simulink model "a8_real_control_smc"  (R2023b)
settings: Solver=FixedStepAuto  StartTime=0.0  StopTime=inf  RelTol=1e-3
undefined symbols (not defined in the file): dev, Main, pid_y_i, pwm_output0
libraries: simulink x15, slpidlib x6, px4Sensorslib x5, px4lib x1, px4uORBlib x1
(part 2 of 2)

== system a8_real_control_smc/RC_cmd/RC2FlightMode/If Action Subsystem2 ==
  In1 : Inport
  Action Port : ActionPort  ActionPortLabel=else
  Out1 : Outport
  wires:
  In1/1 -> Out1/1

== matlab function a8_real_control_smc/Subsystem2/MATLAB Function4 ==
  data: dt input; e_psi input double; u4 output double; e_psi_dot input double; psi_des_dotdot input; s_psi_integ input; phi_dot input; theta_dot input; psi_dot input; reset input; s output; s_psi_integ output
function [u4, s, s_psi_integ] = u4fcn(dt, e_psi, e_psi_dot, psi_des_dotdot,...
                    s_psi_integ, phi_dot, theta_dot, psi_dot, reset)

if (reset == 1); s_psi_integ = 0; end
m = 0.67; g = 9.80665; Ix = 0.0035; Iy = 0.0035; Iz = 0.0069; L = 0.25 / 2;
Kpsi = 0;

alpha = 2;beta = 1;gamma = 0.4;
mu = 25/17;r = 1.5;
K = 5; K1 = 1.5; K2 = 1;

s = alpha * e_psi +  real(beta * sign(e_psi_dot) * (abs(e_psi_dot)) ^ mu) + real(gamma * sign(e_psi) * (abs(e_psi)) ^ r);
s_psi_integ = s_psi_integ + K2 * sign(s) * dt;
s_integ_max = 2;
if s_psi_integ > s_integ_max
    s_psi_integ = s_integ_max;
elseif s_psi_integ < -s_integ_max
    s_psi_integ = -s_integ_max;
end

u4 = -Iz*((Ix-Iy)/Iz*phi_dot*theta_dot - Kpsi/Iz*psi_dot - psi_des_dotdot + alpha/(beta*mu)*sign(e_psi_dot) * (abs(e_psi_dot))^(2-mu)...
    + gamma*r/(beta*mu)*(sign(e_psi) * (abs(e_psi))^(r-1))* sign(e_psi_dot) * (abs(e_psi_dot))^(2-mu) + K1*(abs(s))^(1/2)*sign(s)...
    + s_psi_integ);
u4 = u4 * K;

== matlab function a8_real_control_smc/Subsystem2/MATLAB Function1 ==
  data: dt input; e_theta input double; u3 output double; e_theta_dot input double; theta_des_dotdot input; s_theta_integ input; phi_dot input; theta_dot input; psi_dot input; reset input; s output; s_theta_integ output
function [u3, s, s_theta_integ] = u3fcn(dt, e_theta, e_theta_dot, theta_des_dotdot,...
                    s_theta_integ, phi_dot, theta_dot, psi_dot, reset)

if (reset == 1); s_theta_integ = 0; end
m = 0.67; g = 9.80665; Ix = 0.0035; Iy = 0.0035; Iz = 0.0069; L = 0.25 / 2;
Ktheta = 0;

alpha = 2;beta = 1;gamma = 0.4;
mu = 27/17;r = 1.5;
K1 = 1.5; K2 = (K1^2)/2;

s = alpha * e_theta +  (beta * sign(e_theta_dot) * (abs(e_theta_dot)) ^ mu) + (gamma * sign(e_theta) * (abs(e_theta)) ^ r);
s_theta_integ = s_theta_integ + K2 * sign(s) * dt;
s_integ_max = 2;
if s_theta_integ > s_integ_max
    s_theta_integ = s_integ_max;
elseif s_theta_integ < -s_integ_max
    s_theta_integ = -s_integ_max;
end

u3 = -Iy*((Iz-Ix)/Iy*phi_dot*psi_dot - Ktheta/Iy*theta_dot - theta_des_dotdot + alpha/(beta*mu)*sign(e_theta_dot) * (abs(e_theta_dot))^(2-mu)...
    + gamma*r/(beta*mu)*(sign(e_theta) * (abs(e_theta))^(r-1))* sign(e_theta_dot) * (abs(e_theta_dot))^(2-mu) + K1*(abs(s))^(1/2)*sign(s)...
    + s_theta_integ);

== matlab function a8_real_control_smc/quat2eul ==
  data: q input; phi output; theta output; psi output
function [phi,theta,psi] = quat2eul(q)

% Quaternion conversion to Euler angles based on the PX4 Firmware v1.10.2
% release.

phi = atan2(2*(q(1)*q(2) + q(3)* q(4)), q(1)^2 - q(2)^2 - q(3)^2 + q(4)^2);
theta = asin(-2*(q(2)*q(4) - q(1)*q(3)));
psi = atan2(2*(q(2)*q(3) + q(1)* q(4)), q(1)^2 + q(2)^2 - q(3)^2 - q(4)^2);

end

== matlab function a8_real_control_smc/Subsystem1/MATLAB Function1 ==
  data: phi input double; gain output double; theta input double
function gain = fcn(phi, theta)

gain = 1/(cos(phi) * cos(theta));

== matlab function a8_real_control_smc/Subsystem2/MATLAB Function2 ==
  data: dt input; e_phi input double; u2 output double; e_phi_dot input double; phi_des_dotdot input; s_phi_integ input; phi_dot input; theta_dot input; psi_dot input; s_integ_max input; alpha input; beta input; gamma input; mu input; r input; K1 input; K2 input; reset input; s output; s_phi_integ output
function [u2, s, s_phi_integ] = u2fcn(dt, e_phi, e_phi_dot, phi_des_dotdot,...
                    s_phi_integ, phi_dot, theta_dot, psi_dot, s_integ_max, ...
                    alpha, beta, gamma, mu ,r , K1, K2, reset)

if (reset == 1); s_phi_integ = 0; end
m = 0.67; g = 9.80665; Ix = 0.0035; Iy = 0.0035; Iz = 0.0069; L = 0.25 / 2;
Kphi = 0;

%alpha = 2;beta = 1;gamma = 0.4;
%mu = 15/17;r = 1.1;
%K1 = 1.5; K2 = (K1^2)/2;

s = alpha * e_phi +  (beta * sign(e_phi_dot) * (abs(e_phi_dot)) ^ mu) + (gamma * sign(e_phi) * (abs(e_phi)) ^ r);
s_phi_integ = s_phi_integ + K2 * sign(s) * dt;
if s_phi_integ > s_integ_max
    s_phi_integ = s_integ_max;
elseif s_phi_integ < -s_integ_max
    s_phi_integ = -s_integ_max;
end

u2 = -Ix*((Iy-Iz)/Ix*theta_dot*psi_dot - Kphi/Ix*phi_dot - phi_des_dotdot + alpha/(beta*mu)*sign(e_phi_dot) * (abs(e_phi_dot))^(2-mu)...
    + gamma*r/(beta*mu)*(sign(e_phi) * (abs(e_phi))^(r-1))* sign(e_phi_dot) * (abs(e_phi_dot))^(2-mu) + K1*(abs(s))^(1/2)*sign(s)...
    + s_phi_integ);

== matlab function a8_real_control_smc/fai_d&psi_dGenerator2 ==
  data: psi input double; phi_d output double; u1x input double; u1y input double; u1z input double; theta_d output double
function [phi_d, theta_d] = fcn(psi, u1x, u1y, u1z)

% fai_d = atan((y_d - y)/(x_d - x));
% theta_d = atan((z_d - z)/(((x_d - x)^2 + (y_d - y)^2)^(1/2)));
phi_d = -1 * atan((u1x * sin(psi) - u1y * cos(psi)) / u1z );
theta_d = -1 * atan((u1x * cos(psi) + u1y * sin(psi)) * cos(phi_d) / u1z );

== matlab function a8_real_control_smc/fai_d&psi_dGenerator3 ==
  data: u1 input double; F1 output double; u2 input double; u3 input double; u4 input double; F2 output double; F3 output; F4 output
function [F1,F2,F3,F4] = fcn(u1, u2, u3, u4)

L = 0.25; 
convertMatrix = [1              1           1           1;
                 -L/sqrt(2)     L/sqrt(2)   L/sqrt(2)   -L/sqrt(2);
                 L/sqrt(2)      -L/sqrt(2)  L/sqrt(2)   -L/sqrt(2);
                 0.01           0.01        -0.01       -0.01];
% Km = 1;
% convertMatrix = [1              1           1           1;
%                  -L/sqrt(2)     L/sqrt(2)   L/sqrt(2)   -L/sqrt(2);
%                  L/sqrt(2)      -L/sqrt(2)  L/sqrt(2)   -L/sqrt(2);
%                  Km/sqrt(2)     Km/sqrt(2)  -Km/sqrt(2) -Km/sqrt(2)];
% convertMatrix_inv=[0.2500   -1.4142    1.4142    0.3536;
%                    0.2500    1.4142   -1.4142    0.3536;
%                    0.2500    1.4142    1.4142   -0.3536;
%                    0.2500   -1.4142   -1.4142   -0.3536]
%F = inv(convertMatrix) * [u1; u2; u3; u4];
F = convertMatrix \ [u1; u2; u3; u4];
F1 = F(1);
F2 = F(2);
F3 = F(3);
F4 = F(4);

% convertMatrix_ref = [-0.3536    0.3536    0.3536   -0.3536;
%                       0.3536   -0.3536    0.3536   -0.3536;
%                       0.2500    0.2500   -0.2500   -0.2500;
%                       0.2500    0.2500    0.2500    0.2500];
% convertMatrix_ref_inv = [-1/sqrt(2)       1/sqrt(2)   1 1;
%                           1/sqrt(2)      -1/sqrt(2)   1 1;
%                           1/sqrt(2)       1/sqrt(2)  -1 1;
%                          -1/sqrt(2)      -1/sqrt(2)  -1 1]
